simulink model "Test_Bit_Demultiplexer_1_to_16"  (Simulink 8.7)
settings: Solver=ode45  StartTime=0.0  StopTime=len  RelTol=1e-3
libraries: commutil2 x3, Bit_Demultiplexers_Lib x1
settings Model: Creator=N  LastModifiedBy=Jozko Mrkvicka
settings DataIOCC: LimitDataPoints=off
settings DebuggingCC: UnderspecifiedInitializationDetection=Simplified  MergeDetectMultiDrivingBlocksExec=error
settings HardwareCC: ProdBitPerPointer=64  ProdLargestAtomicFloat=Float  ProdIntDivRoundTo=Zero  ProdEndianess=LittleEndian  ProdHWDeviceType=Intel->x86-64 (Windows64)
settings ModelReferenceCC: PropagateSignalLabelsOutOfModel=on

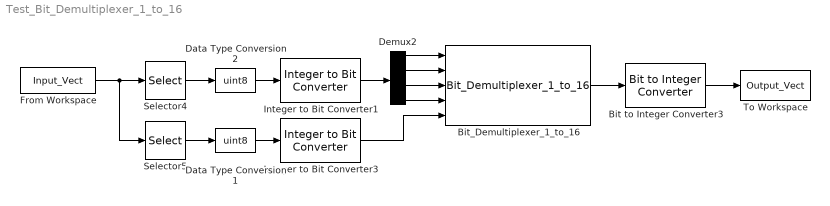
== system Test_Bit_Demultiplexer_1_to_16 ==
  Bit to Integer Converter3 : commutil2/Bit to Integer Converter  nbits=16  bitOrder=MSB first  signedOutputValues=Unsigned  outDtype=uint16  outDtypeSigned=Inherit via internal rule
  Bit_Demultiplexer_1_to_16 : Bit_Demultiplexers_Lib/Bit_Demultiplexers_Lib/Bit_Demultiplexer_1_to_16
  Data Type Conversion1 : DataTypeConversion  OutDataTypeStr=uint8
  Data Type Conversion2 : DataTypeConversion  OutDataTypeStr=uint8
  Demux2 : Demux
  From Workspace : FromWorkspace  VariableName=Input_Vect  SampleTime=1  Interpolate=off  OutputAfterFinalValue=Holding final value
  Integer to Bit Converter1 : commutil2/Integer to Bit Converter  nbits=4  signedInputValues=Unsigned  bitOrder=MSB first  outDtype=uint8
  Integer to Bit Converter3 : commutil2/Integer to Bit Converter  nbits=1  signedInputValues=Unsigned  bitOrder=MSB first  outDtype=uint8
  Selector4 : Selector  IndexMode=Zero-based  InputPortWidth=2  SampleTime=1  IndexOptions=Index vector (dialog)  Indices=0  OutputSizes=1
  Selector5 : Selector  IndexMode=Zero-based  InputPortWidth=2  IndexOptions=Index vector (dialog)  Indices=1  OutputSizes=1
  To Workspace : ToWorkspace  VariableName=Output_Vect  SampleTime=1
  wires:
  Integer to Bit Converter1/1 -> Demux2/1
  Data Type Conversion2/1 -> Integer to Bit Converter1/1
  From Workspace/1 -> Selector5/1, Selector4/1
  Bit_Demultiplexer_1_to_16/1 -> Bit to Integer Converter3/1
  Bit to Integer Converter3/1 -> To Workspace/1
  Selector4/1 -> Data Type Conversion2/1
  Selector5/1 -> Data Type Conversion1/1
  Data Type Conversion1/1 -> Integer to Bit Converter3/1
  Demux2/1 -> Bit_Demultiplexer_1_to_16/1
  Demux2/2 -> Bit_Demultiplexer_1_to_16/2
  Demux2/3 -> Bit_Demultiplexer_1_to_16/3
  Demux2/4 -> Bit_Demultiplexer_1_to_16/4
  Integer to Bit Converter3/1 -> Bit_Demultiplexer_1_to_16/5
